simulink model "impedanceSimulink_updated"  (R2025b)
settings: Solver=VariableStepAuto  StartTime=0.0  StopTime=10.0  RelTol=1e-3
undefined symbols (not defined in the file or in its folder): DH_Parameters
settings Model: Creator=jayde  LastModifiedBy=jayde

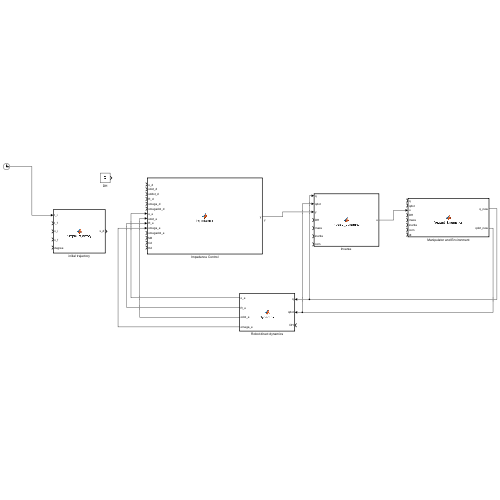
[thumbnail: Simulink's stored preview of the top-level diagram]
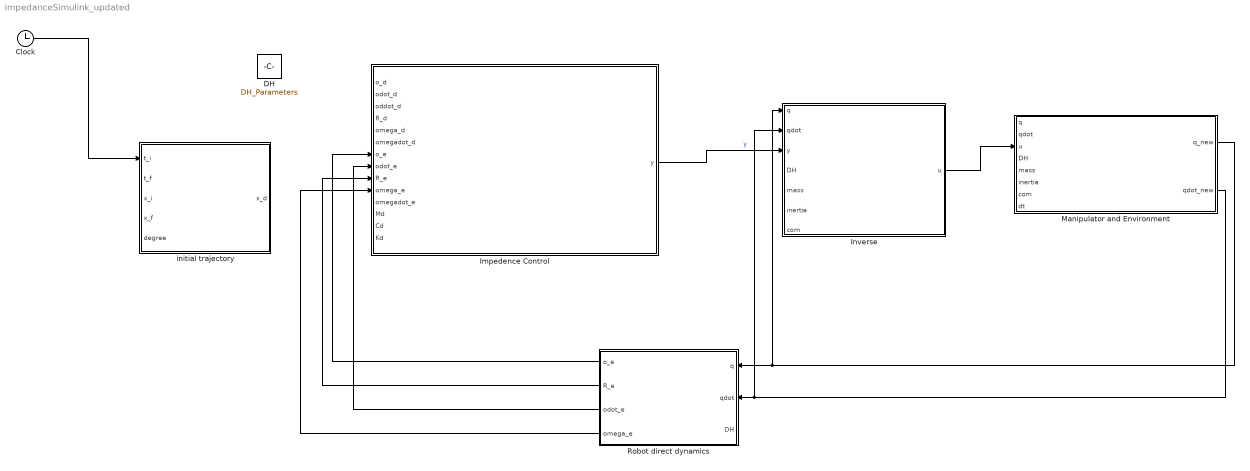
== system impedanceSimulink_updated ==
  Clock : Clock
  DH : Constant  Value=DH_Parameters
  Impedence Control : MATLAB Function  TreatAsAtomicUnit=on
  "Inverse " : MATLAB Function  TreatAsAtomicUnit=on
  Manipulator and Environment : MATLAB Function  TreatAsAtomicUnit=on
  Robot direct dynamics : MATLAB Function  TreatAsAtomicUnit=on
  initial trajectory : MATLAB Function  TreatAsAtomicUnit=on
  wires:
  Clock/1 -> initial trajectory/1(t_i)
  Impedence Control/1(y) -> "Inverse "/3(y)  "y"
  "Inverse "/1(u) -> Manipulator and Environment/3(u)
  Manipulator and Environment/1(q_new) -> "Inverse "/1(q), Robot direct dynamics/1(q)
  Manipulator and Environment/2(qdot_new) -> "Inverse "/2(qdot), Robot direct dynamics/2(qdot)
  Robot direct dynamics/1(o_e) -> Impedence Control/7(o_e)
  Robot direct dynamics/2(R_e) -> Impedence Control/9(R_e)
  Robot direct dynamics/3(odot_e) -> Impedence Control/8(odot_e)
  Robot direct dynamics/4(omega_e) -> Impedence Control/10(omega_e)

== matlab function impedanceSimulink_updated/Manipulator and Environment ==
  data: q input; qdot input; u input; q_new output; DH input; mass input; inertia input; com input; dt input; qdot_new output
function [q_new, qdot_new] = forward_kinematics(q, qdot, u, DH, mass, inertia, com, dt)

[T_all, ~] = fk(q, DH);
n = length(q);

M = Inertial(q, DH, T_all, mass, inertia, com, n);
C = coriolis(q, qdot, DH, mass, inertia, com, n);
G = gravity(q, DH, T_all, mass, com, n);

qddot = M \ (u - C - G);
qdot_new = qdot + qddot*dt;
q_new = q + qdot*dt;
end


function T = dh(a, alpha, d, theta)
    ct = cos(theta);
    st = sin(theta);
    ca = cos(alpha);
    sa = sin(alpha);
    T = [ct, -st*ca, st*sa, a*ct;
         st, ct*ca, -ct*sa, a*st;
         0,     sa,     ca,    d;
         0, 0, 0, 1];
end


function [T_all, o_e] = fk(q, DH)
    n = length(q);
    T = eye(4);
    T_all = zeros(4,4,n);
    for i=1:n
        T = T*dh(DH(i,1), DH(i,2), DH(i,3), q(i)+DH(i,4));
        T_all(:,:,i) = T;
    end
    o_e = T(1:3,4);
end

function M = Inertial_fk(T_all, mass, inertia, com, n)
     M = zeros(n,n);
    for k = 1:n
        J_k = zeros(6,n);
        T_k = T_all(:,:,k);
        R_k = T_K(1:3, 1:3);
        o_k = T_k(1:3,4) + R_k*com(k,:)';

        for  i = 1:k
            if i == 1
                z = [0;0;1]; 
                o = [0;0;0];
            else
                z = T_all(1:3, 3, i-1);
                o = T_all(1:3, 4, i-1);
            end
            J_k(1:3,i) = cross(z, o_k - o);
            J_k(4:6,i) = z;
        end

        I_k = R_k*squeeze(inertia(k,:,:)) * R_k';
        Jv = J_k(1:3,:);
        Jw = J_k(4:6,:);
        M = M + mass(k) * (Jv'*Jv) + Jw'*I_k*Jw;
    end
end

function C = coriolis_fk(q, DH, mass, inertia, com, n)
    dq = 1e-7;
    C = zeros(n,1);
    T_all_nom = fk_c_fk(q, DH, n);
    M_nom = Inertial_fk(q, DH, T_all_nom, mass, inertia, com, n);

    for k = 1:n
        q_p = q; q_p(k) = q_p(k) + dq;
        T_all_p = fk_all_frames_out(q_p, DH, n);
        M_p = Inertial_fk(q_p, DH, T_all_p, mass, inertia, com, n);
        dM  = (M_p - M_nom) / dq;

        C = C + (dM - 0.5*dM') * q_dot * q_dot(k);
    end
    C = 0.5*C;
end

function T_all = fk_c_fk(q, DH)
    T = eye(4);
    T_all = zeros(4,4,n);
     for i=1:n
        T = T*dh(DH(i,1), DH(i,2), DH(i,3), q(i)+DH(i,4));
        T_all(:,:,i) = T;
     end
end

== matlab function impedanceSimulink_updated/Robot direct dynamics ==
  data: o_e output; R_e output; odot_e output; q input; qdot input; DH input; omega_e output
function [o_e, R_e, odot_e, omega_e] = dynamics(q, qdot, DH)

    n = length(q);
    T_all = zeros(4,4,n);

    for i=1:n
        a = DH(i,1);
        alpha = DH(i,2);
        d = DH(i,3);
        theta = q(i) + DH(i, 4);
        Ti = dh(a, alpha, d, theta);
        T = T*Ti;
        T_all(:,:,1) = T;
    end
    R_e = T(1:3, 1:3);
    o_e = T(1:3, 4);
    J = Jacobian2(q, Dh, T_all, o_e);
    V = J*qdot;
    odot_e = V(1:3);
    omega_e = V(4:6);
end



function T = dh(a, alpha, d, theta)
    ct = cos(theta);
    st = sin(theta);
    ca = cos(alpha);
    sa = sin(alpha);
    T = [ct, -st*ca, st*sa, a*ct;
         st, ct*ca, -ct*sa, a*st;
         0,     sa,     ca,    d;
         0, 0, 0, 1];
end

function J = Jacobian2(~, ~, T_all, o_e)
    n = size(T_all, 3);
    J = zeros(6,n);
    for i = 1:n
        if i == 1
            z = [0;0;1]; o = [0;0;0];
        else
            z = T_all(1:3,3,i-1);
            o = T_all(1:3,4,i-1);
        end
        J(1:3,i) = cross(z, o_e - o);
        J(4:6,i) = z;
    end
end

== matlab function impedanceSimulink_updated/Impedence Control ==
  data: o_d input; odot_d input; oddot_d input; R_d input; omega_d input; omegadot_d input; o_e input; odot_e input; y output; R_e input; omega_e input; omegadot_e input; Md input; Cd input; Kd input
function y = impedance(o_d, odot_d,  oddot_d, R_d,...
                                            omega_d, omegadot_d, ...
                                            o_e, odot_e , R_e, ...
                                            omega_e, omegadot_e, ...
                                            Md, Cd, Kd)

e_position = o_d - o_e;
R_e = R_d*R_e';
s = (R_e - R_e') / 2;
e_Rotation = [s(3,2); s(1,3); s(2,1)];
x_error = [e_position, e_Rotation];

e_velocity = odot_d - odot_e;
e_omega = omega_d - omega_e;
xdot_error = [e_velocity, e_omega];

xddot_d = [oddot_d;
           omegadot_d];

% y = [oddot_dref, alpha_ref]
y = xddot_d + Md \ (Cd*xdot_error + Kd*x_error);

end

== matlab function impedanceSimulink_updated/Inverse  ==
  data: q input; u output; qdot input; y input; DH input; mass input; inertia input; com input
function u = inverse_dynamics(q, qdot, y, DH, mass, inertia, com)

n = length(q);
[T_all, ~] = forward_kinematics(q, DH);
J = Jacobian(q, robot);
J_pinv = pinv(J);
qddot_ref = J_pinv * y;

% dynamic forces
M = Inertial(q, DH, T_all, mass, inertia, com, n);
C = coriolis(q, qdot, DH, mass, inertia, com, n);
G = gravity(q, DH, T_all, mass, com, n);

u = M.*qddot_ref + C + G;

end


function T = dh(a, alpha, d, theta)
    ct = cos(theta);
    st = sin(theta);
    ca = cos(alpha);
    sa = sin(alpha);
    T = [ct, -st*ca, st*sa, a*ct;
         st, ct*ca, -ct*sa, a*st;
         0,     sa,     ca,    d;
         0, 0, 0, 1];
end


function [T_all, o_e] = forward_kinematics(q, DH)
    n = length(q);
    T = eye(4);
    T_all = zeros(4,4,n);
    for i=1:n
        T = T*dh(DH(i,1), DH(i,2), DH(i,3), q(i)+DH(i,4));
        T_all(:,:,i) = T;
    end
    o_e = T(1:3,4);
end

function J = Jacobian(~, ~, T_all, o_e, n)
    J = zeros(6,n);
    for i = 1:n
        if i == 1
            z = [0;0;1]; o = [0;0;0];
        else
            z = T_all(1:3,3,i-1);
            o = T_all(1:3,4,i-1);
        end
        J(1:3,i) = cross(z, o_e - o);
        J(4:6,i) = z;
    end
end

function M = Inertial(T_all, mass, inertia, com, n)
     M = zeros(n,n);
    for k = 1:n
        J_k = zeros(6,n);
        T_k = T_all(:,:,k);
        R_k = T_K(1:3, 1:3);
        o_k = T_k(1:3,4) + R_k*com(k,:)';

        for  i = 1:k
            if i == 1
                z = [0;0;1]; 
                o = [0;0;0];
            else
                z = T_all(1:3, 3, i-1);
                o = T_all(1:3, 4, i-1);
            end
            J_k(1:3,i) = cross(z, o_k - o);
            J_k(4:6,i) = z;
        end

        I_k = R_k*squeeze(inertia(k,:,:)) * R_k';
        Jv = J_k(1:3,:);
        Jw = J_k(4:6,:);
        M = M + mass(k) * (Jv'*Jv) + Jw'*I_k*Jw;
    end
end

function C = coriolis(q, DH, mass, inertia, com, n)
    dq = 1e-7;
    C = zeros(n,1);
    T_all_nom = fk_c(q, DH, n);
    M_nom = Inertial(q, DH, T_all_nom, mass, inertia, com, n);

    for k = 1:n
        q_p = q; q_p(k) = q_p(k) + dq;
        T_all_p = fk_all_frames_out(q_p, DH, n);
        M_p = Inertial(q_p, DH, T_all_p, mass, inertia, com, n);
        dM  = (M_p - M_nom) / dq;

        C = C + (dM - 0.5*dM') * q_dot * q_dot(k);
    end
    C = 0.5*C;
end

function G = gravity(T_all, mass, com, n)
    g0 = [0;0;-9.81];
    g = zeros(n,1);
    for k = 1:n
        R_k = T_all(1:3,1:3, k);
        o_k_com = T_all(1:3, 4,k) + R_k*com(k,:)';
        for i = 1:k
             if i == 1
                z = [0;0;1]; 
                o = [0;0;0];
             else
                z = T_all(1:3, 3, i-1);
                o = T_all(1:3, 4, i-1);
             end
             Jv_k = cross(z, o_k_com - o);
             g(i) = g(i) - mass(k) * g0' * Jv_k;
        end
    end
end

%function for corialis that doesn't return error
function T_all = fk_c(q, DH)
    T = eye(4);
    T_all = zeros(4,4,n);
     for i=1:n
        T = T*dh(DH(i,1), DH(i,2), DH(i,3), q(i)+DH(i,4));
        T_all(:,:,i) = T;
     end
end

== matlab function impedanceSimulink_updated/initial trajectory ==
  data: t_i input; x_d output; t_f input; x_i input; x_f input; degree input
function x_d = SimpleTrajectory(t_i, t_f, x_i, x_f, degree)


if degree == 3 || degree == 5   

    if length(x_i) ~= length(x_f)
        disp("Initial and final dimensions aren't the same.")
        return
    end

    dimension = length(x_i);
    
    A = sym('A',[dimension degree+1]);
    P = sym('P', [dimension 1]);
    dP = sym('dP', [dimension 1]);
    
    E = {};
    dE = {};

    P_sol = sym('P_sol', [dimension 1]);
    
    syms t

    if degree == 3
        for i = 1:dimension
            P(i) = A(i, 1);
            dP(i) = 0;
        
            for j=2:degree+1
                P(i) = P(i) + A(i, j)*(t)^(j-1);
                dP(i) = diff(P(i), t);
            end
        
            E{i} = [subs(P(i), t, t_i) == x_i(i), subs(P(i), t, t_f) == x_f(i)];
            dE{i} = [subs(dP(i), t, t_i) == 0, subs(dP(i), t, t_f) == 0];
        
            sol = solve([E{i}, dE{i}], A(i, :));
        
            A_sol = cell2mat(struct2cell(sol))';
            P_sol(i) = subs(P(i), A(i, :), A_sol);    
        end

    

    else
        d2P = sym('d2P', [dimension 1]);
        d2E = {};

        for i = 1:dimension
            P(i) = A(i, 1);
            dP(i) = 0;
            d2P(i) = 0;
        
            for j=2:degree+1
                P(i) = P(i) + A(i, j)*(t)^(j-1);
                dP(i) = diff(P(i), t);
                d2P(i) = diff(P(i), t, 2);
            end
        
            E{i} = [subs(P(i), t, t_i) == x_i(i), subs(P(i), t, t_f) == x_f(i)];
            dE{i} = [subs(dP(i), t, t_i) == 0, subs(dP(i), t, t_f) == 0];
            d2E{i} = [subs(d2P(i), t, t_i) == 0, subs(d2P(i), t, t_f) == 0];
        
            sol = solve([E{i}, dE{i}, d2E{i}], A(i, :));
        
            A_sol = cell2mat(struct2cell(sol))';
            P_sol(i) = subs(P(i), A(i, :), A_sol);    
        end
    end

x_d = P_sol;

else
    disp("Degree must be 3 or 5")
end

end
